simulink model "TorqueTransitionHandler"  (R2016b)
settings: Solver=FixedStepAuto  StartTime=0.0  StopTime=10.0  FixedStep=0.002  RelTol=1e-3  EnableMultiTasking=on
settings Model: Creator=march  LastModifiedBy=snyke7
settings SolverCC: EnableConcurrentExecution=on
settings DataIOCC: SaveFormat=StructureWithTime
settings OptimizationCC: BlockReduction=off  OptimizeBlockIOStorage=off  BufferReuse=off  GlobalBufferReuse=off  ExpressionFolding=off  LocalBlockOutputs=off
settings HardwareCC: ProdBitPerPointer=32  ProdBitPerSizeT=32  ProdBitPerPtrDiffT=32  ProdLargestAtomicFloat=None  ProdWordSize=32  ProdLongLongMode=on  ProdHWDeviceType=Generic->32-bit x86 compatible
settings RTWCC: SystemTargetFile=slrt.tlc  TemplateMakefile=slrt_default_tmf  Description=Simulink Real-Time  RTWCompilerOptimization=on
settings TargetCC: CodeReplacementLibrary=XPC_BLAS  ParMdlRefBuildCompliant=on  ConcurrentExecutionCompliant=on  GeneratePreprocessorConditionals=Use local settings  MatFileLogging=on  MATLABClassNameForMDSCustomization=xpcAperiodicCustomization

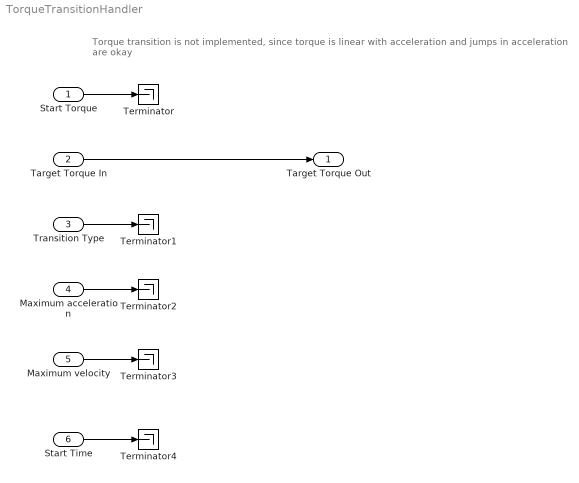
== system TorqueTransitionHandler ==
  note: Torque transition is not implemented, since torque is linear with acceleration and jumps in acceleration are okay
  Start Torque : Inport
  Target Torque In : Inport  Port=2
  Transition Type : Inport  Port=3
  Maximum acceleration : Inport  Port=4
  Maximum velocity : Inport  Port=5
  Start Time : Inport  Port=6
  Terminator{,1..4} (5 alike) : Terminator
  Target Torque Out : Outport
  wires:
  Target Torque In/1 -> Target Torque Out/1
  Start Torque/1 -> Terminator/1
  Transition Type/1 -> Terminator1/1
  Maximum acceleration/1 -> Terminator2/1
  Maximum velocity/1 -> Terminator3/1
  Start Time/1 -> Terminator4/1
